simulink model "interlvrdoc"  (Simulink 5.0)
settings: Solver=ode45  SolverMode=SingleTasking  StartTime=0.0  StopTime=length(errors)  RelTol=1e-3
undefined symbols (not defined in the file or in its folder): gfprimfd, slcm
libraries: dspbuff3 x2, commblkcod2 x2, commblkintrlv2 x2, commsource2 x1, commsink2 x1, dspsrcs4 x1
settings Model: Creator=ptrow  LastModifiedBy=ptrow  SaveTime=off  SaveOutput=off  AlgebraicLoopMsg=error  RTWOptions=-aRollThreshold=5  RTWInlineParameters=on  BooleanDataType=off

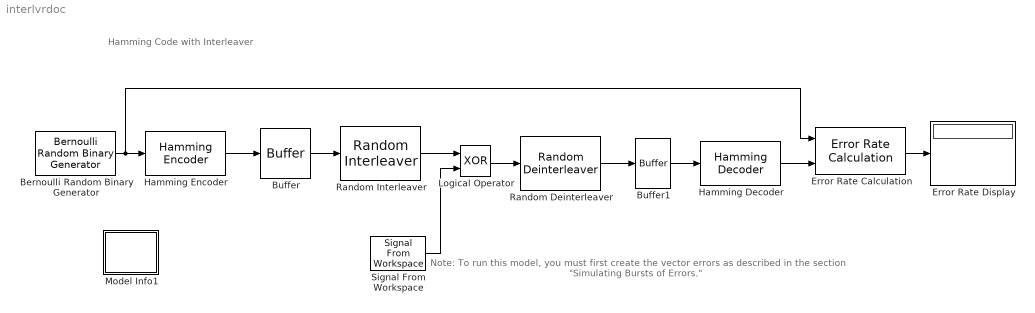
== system interlvrdoc ==
  note: Hamming Code with Interleaver
  note: Note: To run this model, you must first create the vector errors
      | as described in the section "Simulating Bursts of Errors."
  Bernoulli Random Binary Generator : commsource2/Bernoulli Random Binary Generator  P=0.5  seed=435345  Ts=1  frameBased=on  sampPerFrame=4  orient=off
  Buffer : dspbuff3/Buffer  N=84  V=0  ic=0
  Buffer1 : dspbuff3/Buffer  N=7  V=0  ic=0
  Error Rate Calculation : commsink2/Error Rate Calculation  N=(4/7)*84  st_delay=100  cp_mode=Entire frame  subframe=[]  PMode=Port  WsName=ErrorVec  RsMode2=off  stop=off  numErr=100  maxBits=1000
  Error Rate Display : Display
      settings: Format=short
  Hamming Decoder : commblkcod2/Hamming Decoder  n=7  k=gfprimfd(3,'min')
  Hamming Encoder : commblkcod2/Hamming Encoder  n=7  k=gfprimfd(3,'min')
  Logical Operator : Logic  Operator=XOR  Inputs=2
  Model Info1 : Subsystem  LoadFcn=slcm LoadBlock;  InitFcn=slcm('UpdateAllCMBlocksInThisModelInit')  mask(CMBlock){InitialSaveTempField=, InitialBlockCM=None, BlockCM=None, Frame=on, SaveTempField=, DisplayStringWithTags=Info, MaskDisplayString=Info, HorizontalTextAlignment=Center, LeftAlignmentValue=0.5, SourceBlockDiagram=interlvrdoc, TagMaxNumber=20, CMTag1=, CMTag2=, CMTag3=, CMTag4=, CMTag5=, CMTag6=, CMTag7=, CMTag8=, CMTag9=, CMTag10=, CMTag11=, CMTag12=, CMTag13=, CMTag14=, CMTag15=, CMTag16=, CMTag17=, CMTag18=, CMTag19=, CMTag20=}
      mask help: This block allows revision control information to be displayed within the model.
      settings: CopyFcn=slcm CopyBlock;  DeleteFcn=slcm Cancel;  PostSaveFcn=slcm('UpdateAllCMBlocksInThisModel')  NameChangeFcn=slcm Rename;  OpenFcn=commdemohelp;  RTWFcnNameOpts=Auto  RTWFileNameOpts=Auto
      mask Display: text(str2num(LeftAlignmentValue), 0.5, MaskDisplayString, 'HorizontalAlignment', HorizontalTextAlignment)
  Random Deinterleaver : commblkintrlv2/Random Deinterleaver  N=84  seed=113
  Random Interleaver : commblkintrlv2/Random Interleaver  N=84  seed=113
  Signal From Workspace : dspsrcs4/Signal From Workspace  X=errors  Ts=4/7  nsamps=84  OutputAfterFinalValue=Setting to zero
  wires:
  Error Rate Calculation/1 -> Error Rate Display/1
  Hamming Decoder/1 -> Error Rate Calculation/2
  Hamming Encoder/1 -> Buffer/1
  Buffer/1 -> Random Interleaver/1
  Buffer1/1 -> Hamming Decoder/1
  Random Deinterleaver/1 -> Buffer1/1
  Random Interleaver/1 -> Logical Operator/1
  Logical Operator/1 -> Random Deinterleaver/1
  Bernoulli Random Binary Generator/1 -> Hamming Encoder/1, Error Rate Calculation/1
  Signal From Workspace/1 -> Logical Operator/2

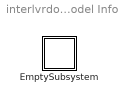
== system interlvrdoc/Model Info1 ==
  EmptySubsystem : Subsystem
      settings: RTWFcnNameOpts=Auto  RTWFileNameOpts=Auto

== system interlvrdoc/Model Info1/EmptySubsystem ==
